simulink model "Simulacion_stepper"  (R2025b)
settings: Solver=ode4  StartTime=0.0  StopTime=Time_simulation  FixedStep=1/frecuency_simulation  RelTol=1e-3
InitFcn:
  | %%InitFcn();
StopFcn:
  | %%FinishFcn
model workspace (MAT data in the model file):
  Ts_stepper = 0.001
values from neighbouring files (symbols this model uses):
  B = motor_params.B_internal    [bode.m]    (also in current_observer.m = 0.0005; discretizacion.m = [ 1/L, 0; ekf_4_estados.m = params.B; obs_ctrl_back_emf_ext.m = [1/L 0)
  frecuency_simulation = 10e3    (= 10000)    [InitFcn.m]
  J = motor_params.J_internal    [bode.m]    (also in current_observer.m = 0.008; ekf_4_estados.m = params.J; obs_ctrl_back_emf_ext.m = 0.008; obs_y_contrl_back_emd.m = 0.008)
  Ke = 0.0055    [current_observer.m]    (also in ekf_4_estados.m = params.Ke; observer.m = Pvec(3); salient_motor.m = 0.0066)
  Ki_d = PI_dq_params.Ki_d_salient    [bode.m]
  Ki_q = PI_dq_params.Ki_q_salient    [bode.m]
  Ki_w = (wn_w^2)*J_var/Kt    [Barrido_B.m]    (also in Barrido_J.m; bode.m = PI_MTPA_params.Ki_w)
  Kp_d = PI_dq_params.Kp_d_salient    [bode.m]
  Kp_q = PI_dq_params.Kp_q_salient    [bode.m]
  Kp_w = (2*shi_w*wn_w*J_var)/Kt    [Barrido_B.m]    (also in Barrido_J.m; bode.m = PI_MTPA_params.Kp_w)
  Kt = Nr*Ke    (= 0.275)    [current_observer.m]    (also in ekf_4_estados.m = params.Kt; frecuencia_max.m = 0.33; observer.m = Pvec(4); salient_motor.m = 0.33)
  L = place(A', C', 10*eig(A)).'    [current_observer.m]    (also in desfase.m = lags(k); discretizacion.m = 0.01; frecuencia_max.m = 0.006; obs_ctrl_back_emf_ext.m = 0.006)
  P = motor_params.P    [bode.m]    (also in ekf_4_estados.m = P_pred; frecuencia_max.m = 50; salient_motor.m = 50)
  R = motor_params.R    [bode.m]    (also in current_observer.m = 3.4; discretizacion.m = 3.4; ekf_4_estados.m = params.R; frecuencia_max.m = 3.4)
  sample_time = 1/frecuency_simulation    (= 0.0001)    [InitFcn.m]
  Ts_current = 1/f_current    (= 0.0001)    [InitFcn.m]
  Ts_Wm = Ts_current*10    (= 0.001)    [InitFcn.m]
  Vdc = 24    [InitFcn.m]    (also in frecuencia_max.m = 12)
undefined symbols (not defined in the file or in its folder): DiscIntNeverNeededParam, EKF_params, motor_params, RI_base
libraries: simulink x8, mcbeeMathTransformLib x3, spspowerguiLib x1
(part 2 of 5)

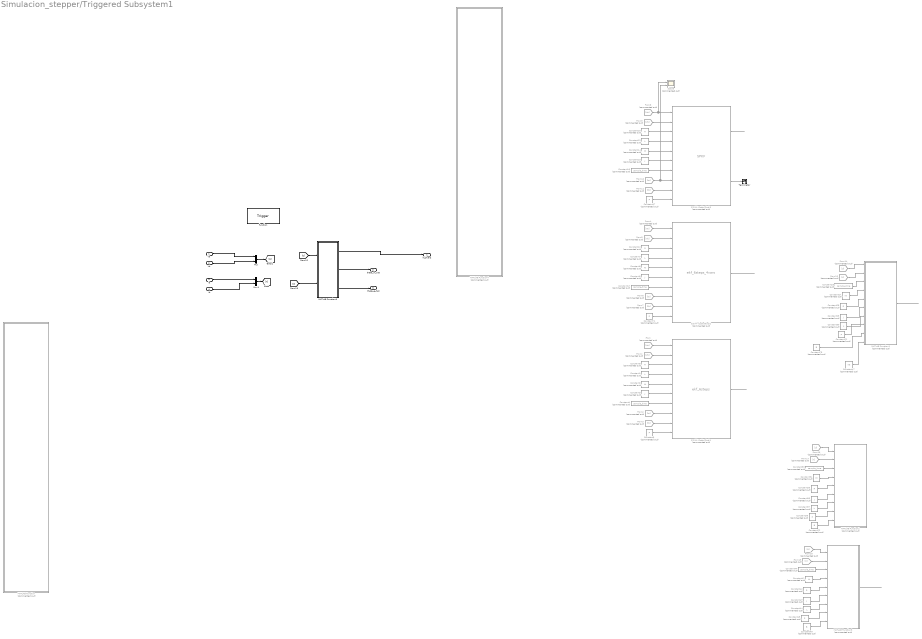
== system Simulacion_stepper/Triggered Subsystem1 ==
  Va : Inport
  Vb : Inport  Port=2
  Ia : Inport  Port=3
  Ib : Inport  Port=4
  function : TriggerPort  TriggerType=function-call  VariantControl=(inherit)  SampleTime=1/100
  C/C++ Code Block1 : S-Function  Commented=on  FunctionName=ekf_6steps  SFunctionModules=ekf_6steps_wrapper.c  SFunctionDeploymentMode=off  EnableBusSupport=off  mask(S-Function Builder){}
      mask help: Simulink:masks:SFunctionBuilder_MD
      mask init: same as Simulacion_stepper/Motor 1  Speed PR/C/C++ Code Block
      settings: CopyFcn=set_param(gcbh,'LinkStatus','none')  OpenFcn=sfunctionwizard(gcbh)
      mask Display:
      | plot(val(:,1),val(:,2))
      | disp(sys)
      | port_label('input',1,sprintf('%s', 'Va'),'interpreter','tex')
      | port_label('input',2,sprintf('%s', 'Vb'),'interpreter','tex')
      | port_label('input',3,sprintf('%s', 'R'),'interpreter','tex')
      | port_label('input',4,sprintf('%s', 'L'),'interpreter','tex')
      | port_label('input',5,sprintf('%s', 'Kt'),'interpreter','tex')
      | port_label('input',6,sprintf('%s', 'J'),'interpreter','tex')
      | port_label('input',7,sprintf('%s', 'Ts'),'interpreter','tex')
      | port_label('input',8,sprintf('%s', 'Ia\_medido'),'interpreter','tex')
      | port_label('input',9,sprintf('%s', 'Ib\_medido'),'interpreter','tex')
      | port_label('input',10,sprintf('%s', 'Nr'),'interpreter','tex')
      | port_label('output',1,sprintf('%s', 'x\_corr\_out'),'interpreter','tex')
  C/C++ Code Block2 : S-Function  Commented=on  FunctionName=ekf_6steps_4vars  SFunctionModules=ekf_6steps_4vars_wrapper.c  SFunctionDeploymentMode=off  EnableBusSupport=off  mask(S-Function Builder){}
      mask help: Simulink:masks:SFunctionBuilder_MD
      mask init: same as Simulacion_stepper/Motor 1  Speed PR/C/C++ Code Block
      settings: CopyFcn=set_param(gcbh,'LinkStatus','none')  OpenFcn=sfunctionwizard(gcbh)
      mask Display:
      | plot(val(:,1),val(:,2))
      | disp(sys)
      | port_label('input',1,sprintf('%s', 'Va'),'interpreter','tex')
      | port_label('input',2,sprintf('%s', 'Vb'),'interpreter','tex')
      | port_label('input',3,sprintf('%s', 'R'),'interpreter','tex')
      | port_label('input',4,sprintf('%s', 'L'),'interpreter','tex')
      | port_label('input',5,sprintf('%s', 'Kt'),'interpreter','tex')
      | port_label('input',6,sprintf('%s', 'J'),'interpreter','tex')
      | port_label('input',7,sprintf('%s', 'Ts'),'interpreter','tex')
      | port_label('input',8,sprintf('%s', 'Ia\_medido'),'interpreter','tex')
      | port_label('input',9,sprintf('%s', 'Ib\_medido'),'interpreter','tex')
      | port_label('input',10,sprintf('%s', 'Nr'),'interpreter','tex')
      | port_label('output',1,sprintf('%s', 'x\_corr\_out'),'interpreter','tex')
  C/C++ Code Block3 : S-Function  Commented=on  FunctionName=SPKF  SFunctionModules=SPKF_wrapper.c  SFunctionDeploymentMode=off  EnableBusSupport=off  mask(S-Function Builder){}
      mask help: Simulink:masks:SFunctionBuilder_MD
      mask init: same as Simulacion_stepper/Motor 1  Speed PR/C/C++ Code Block
      settings: CopyFcn=set_param(gcbh,'LinkStatus','none')  OpenFcn=sfunctionwizard(gcbh)
      mask Display:
      | plot(val(:,1),val(:,2))
      | disp(sys)
      | port_label('input',1,sprintf('%s', 'Va'),'interpreter','tex')
      | port_label('input',2,sprintf('%s', 'Vb'),'interpreter','tex')
      | port_label('input',3,sprintf('%s', 'R'),'interpreter','tex')
      | port_label('input',4,sprintf('%s', 'L'),'interpreter','tex')
      | port_label('input',5,sprintf('%s', 'Kt'),'interpreter','tex')
      | port_label('input',6,sprintf('%s', 'J'),'interpreter','tex')
      | port_label('input',7,sprintf('%s', 'Ts'),'interpreter','tex')
      | port_label('input',8,sprintf('%s', 'Ia\_medido'),'interpreter','tex')
      | port_label('input',9,sprintf('%s', 'Ib\_medido'),'interpreter','tex')
      | port_label('input',10,sprintf('%s', 'Nr'),'interpreter','tex')
      | port_label('output',1,sprintf('%s', 'x'),'interpreter','tex')
      | port_label('output',2,sprintf('%s', 'x\_aux'),'interpreter','tex')
  Constant{1,7,13,30,37,44} (6 alike) : Constant  Commented=on  Value=L  OutDataTypeStr=double
  Constant{4,10,16,26,33,40} (6 alike) : Constant  Commented=on  Value=sample_time  OutDataTypeStr=double
  Constant{5,11,17,31,38,45} (6 alike) : Constant  Commented=on  Value=P  OutDataTypeStr=double
  Constant{6,12,18,28,35,42} (6 alike) : Constant  Commented=on  Value=R  OutDataTypeStr=double
  Constant{2,8,14,27,34,41} (6 alike) : Constant  Commented=on  Value=Kt  OutDataTypeStr=double
  Constant{3,9,15,29,36,43} (6 alike) : Constant  Commented=on  Value=J  OutDataTypeStr=double
  Constant25 : Constant  Commented=on  Value=B
  Constant32 : Constant  Commented=on  Value=B
  Constant39 : Constant  Commented=on  Value=B
  Constant47 : Constant  Commented=on  Value=Ke  OutDataTypeStr=double
  From : From  Commented=on  GotoTag=Va
  From1 : From  Commented=on  GotoTag=Vb
  From10 : From  Commented=on  GotoTag=Ia
  From11 : From  Commented=on  GotoTag=Ib
  From14 : From  Commented=on  GotoTag=U
  From15 : From  Commented=on  GotoTag=X
  From16 : From  Commented=on  GotoTag=U
  From17 : From  Commented=on  GotoTag=X
  From18 : From  Commented=on  GotoTag=U
  From19 : From  Commented=on  GotoTag=X
  From2 : From  Commented=on  GotoTag=Ia
  From3 : From  Commented=on  GotoTag=Ib
  From4 : From  Commented=on  GotoTag=Va
  From5 : From  Commented=on  GotoTag=Vb
  From6 : From  Commented=on  GotoTag=Ia
  From7 : From  Commented=on  GotoTag=Ib
  From8 : From  Commented=on  GotoTag=Va
  From9 : From  Commented=on  GotoTag=Vb
  MATLAB Function : MATLAB Function  Commented=on  TreatAsAtomicUnit=on
  MATLAB Function1 : MATLAB Function  Commented=on  TreatAsAtomicUnit=on
  MATLAB Function2 : MATLAB Function  Commented=on  TreatAsAtomicUnit=on
  MATLAB Function3 : MATLAB Function  Commented=on  TreatAsAtomicUnit=on
  MATLAB Function4 : MATLAB Function  Commented=on  TreatAsAtomicUnit=on
  MATLAB Function5 : MATLAB Function  TreatAsAtomicUnit=on
  Mux : Mux  Inputs=2
  Mux1 : Mux  Inputs=2
  Scope : Scope  Commented=on  NumInputPorts=2
      settings: ActiveDisplayYMinimum=-25.65057  ActiveDisplayYMaximum=25.22013
  Terminator : Terminator
  kf_5var2 : Outport  PortDimensions=[5 1]
  theta_m_hat : Outport  Port=2
  theta_e_hat : Outport  Port=3
  wires:
  Constant4/1 -> C/C++ Code Block1/7
  Constant5/1 -> C/C++ Code Block1/10
  C/C++ Code Block1/1 -> ?
  Constant6/1 -> C/C++ Code Block1/3
  Constant1/1 -> C/C++ Code Block1/4
  Constant2/1 -> C/C++ Code Block1/5
  Constant3/1 -> C/C++ Code Block1/6
  C/C++ Code Block2/1 -> ?
  C/C++ Code Block3/1 -> ?
  Vb/1 -> Mux/2
  Va/1 -> Mux/1
  Ib/1 -> Mux1/2
  Ia/1 -> Mux1/1
  From/1 -> C/C++ Code Block1/1
  From1/1 -> C/C++ Code Block1/2
  From2/1 -> C/C++ Code Block1/8
  From3/1 -> C/C++ Code Block1/9
  From4/1 -> C/C++ Code Block2/1
  From7/1 -> C/C++ Code Block2/9
  Constant8/1 -> C/C++ Code Block2/5
  Constant12/1 -> C/C++ Code Block2/3
  From5/1 -> C/C++ Code Block2/2
  Constant11/1 -> C/C++ Code Block2/10
  From6/1 -> C/C++ Code Block2/8
  Constant9/1 -> C/C++ Code Block2/6
  Constant7/1 -> C/C++ Code Block2/4
  Constant10/1 -> C/C++ Code Block2/7
  From8/1 -> Scope/1, C/C++ Code Block3/1
  From11/1 -> C/C++ Code Block3/9
  Constant14/1 -> C/C++ Code Block3/5
  Constant18/1 -> C/C++ Code Block3/3
  From9/1 -> C/C++ Code Block3/2
  Constant17/1 -> C/C++ Code Block3/10
  From10/1 -> Scope/2, C/C++ Code Block3/8
  Constant15/1 -> C/C++ Code Block3/6
  Constant13/1 -> C/C++ Code Block3/4
  Constant16/1 -> C/C++ Code Block3/7
  C/C++ Code Block3/2 -> Terminator/1
  Mux1/1 -> [X]
  Mux/1 -> [U]
  From16/1 -> MATLAB Function2/1(U)
  From17/1 -> MATLAB Function2/2(Y)
  Constant33/1 -> MATLAB Function2/3(Ts)
  Constant32/1 -> MATLAB Function2/9(B)
  Constant37/1 -> MATLAB Function2/7(L)
  Constant35/1 -> MATLAB Function2/5(R)
  Constant36/1 -> MATLAB Function2/6(J)
  Constant34/1 -> MATLAB Function2/4(Kt)
  Constant38/1 -> MATLAB Function2/8(Nr)
  MATLAB Function3/1(x_corr) -> ?
  Constant45/1 -> MATLAB Function3/8(Nr)
  Constant41/1 -> MATLAB Function3/4(Kt)
  From19/1 -> MATLAB Function3/2(Y)
  Constant43/1 -> MATLAB Function3/6(J)
  Constant40/1 -> MATLAB Function3/3(Ts)
  Constant39/1 -> MATLAB Function3/9(B)
  Constant42/1 -> MATLAB Function3/5(R)
  From18/1 -> MATLAB Function3/1(U)
  Constant44/1 -> MATLAB Function3/7(L)
  From15/1 -> MATLAB Function1/2(X)
  Constant27/1 -> MATLAB Function1/4(Kt)
  Constant31/1 -> MATLAB Function1/8(Nr)
  Constant29/1 -> MATLAB Function1/6(J)
  Constant25/1 -> MATLAB Function1/9(B)
  Constant26/1 -> MATLAB Function1/3(Ts)
  Constant30/1 -> MATLAB Function1/7(L)
  Constant28/1 -> MATLAB Function1/5(R)
  From14/1 -> MATLAB Function1/1(U)
  Constant47/1 -> MATLAB Function1/10(Ke)
  MATLAB Function1/1(x_corr) -> ?
  [X] -> MATLAB Function5/2(X)
  [U] -> MATLAB Function5/1(U)
  MATLAB Function5/1(x_out) -> kf_5var2/1
  MATLAB Function5/2(theta_m_hat) -> theta_m_hat/1
  MATLAB Function5/3(theta_e_out) -> theta_e_hat/1

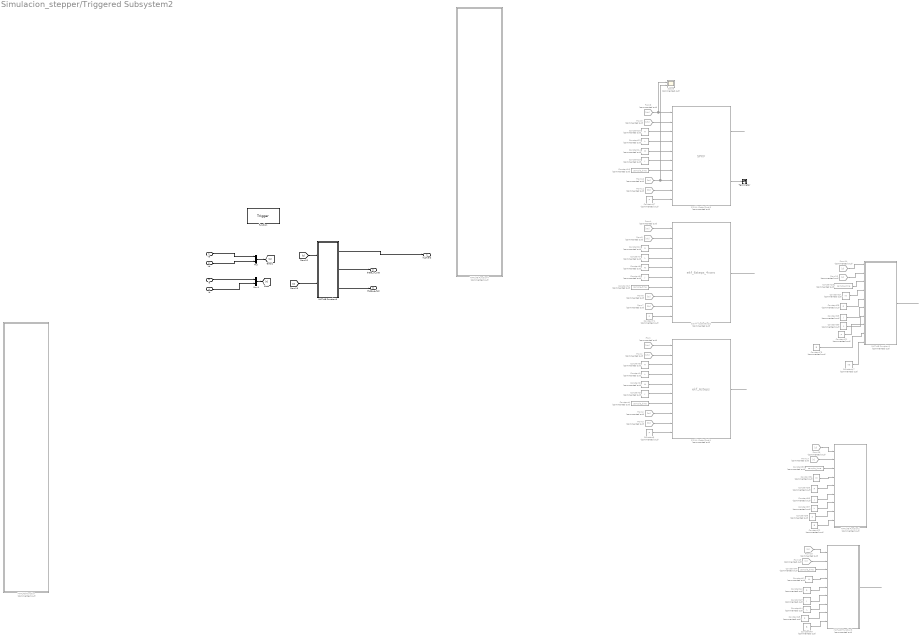
== system Simulacion_stepper/Triggered Subsystem2 ==
  Va : Inport
  Vb : Inport  Port=2
  Ia : Inport  Port=3
  Ib : Inport  Port=4
  function : TriggerPort  TriggerType=function-call  VariantControl=(inherit)  SampleTime=1/100
  C/C++ Code Block1 : S-Function  Commented=on  FunctionName=ekf_6steps  SFunctionModules=ekf_6steps_wrapper.c  SFunctionDeploymentMode=off  EnableBusSupport=off  mask(S-Function Builder){}
      mask help: Simulink:masks:SFunctionBuilder_MD
      mask init: same as Simulacion_stepper/Motor 1  Speed PR/C/C++ Code Block
      settings: CopyFcn=set_param(gcbh,'LinkStatus','none')  OpenFcn=sfunctionwizard(gcbh)
      mask Display:
      | plot(val(:,1),val(:,2))
      | disp(sys)
      | port_label('input',1,sprintf('%s', 'Va'),'interpreter','tex')
      | port_label('input',2,sprintf('%s', 'Vb'),'interpreter','tex')
      | port_label('input',3,sprintf('%s', 'R'),'interpreter','tex')
      | port_label('input',4,sprintf('%s', 'L'),'interpreter','tex')
      | port_label('input',5,sprintf('%s', 'Kt'),'interpreter','tex')
      | port_label('input',6,sprintf('%s', 'J'),'interpreter','tex')
      | port_label('input',7,sprintf('%s', 'Ts'),'interpreter','tex')
      | port_label('input',8,sprintf('%s', 'Ia\_medido'),'interpreter','tex')
      | port_label('input',9,sprintf('%s', 'Ib\_medido'),'interpreter','tex')
      | port_label('input',10,sprintf('%s', 'Nr'),'interpreter','tex')
      | port_label('output',1,sprintf('%s', 'x\_corr\_out'),'interpreter','tex')
  C/C++ Code Block2 : S-Function  Commented=on  FunctionName=ekf_6steps_4vars  SFunctionModules=ekf_6steps_4vars_wrapper.c  SFunctionDeploymentMode=off  EnableBusSupport=off  mask(S-Function Builder){}
      mask help: Simulink:masks:SFunctionBuilder_MD
      mask init: same as Simulacion_stepper/Motor 1  Speed PR/C/C++ Code Block
      settings: CopyFcn=set_param(gcbh,'LinkStatus','none')  OpenFcn=sfunctionwizard(gcbh)
      mask Display:
      | plot(val(:,1),val(:,2))
      | disp(sys)
      | port_label('input',1,sprintf('%s', 'Va'),'interpreter','tex')
      | port_label('input',2,sprintf('%s', 'Vb'),'interpreter','tex')
      | port_label('input',3,sprintf('%s', 'R'),'interpreter','tex')
      | port_label('input',4,sprintf('%s', 'L'),'interpreter','tex')
      | port_label('input',5,sprintf('%s', 'Kt'),'interpreter','tex')
      | port_label('input',6,sprintf('%s', 'J'),'interpreter','tex')
      | port_label('input',7,sprintf('%s', 'Ts'),'interpreter','tex')
      | port_label('input',8,sprintf('%s', 'Ia\_medido'),'interpreter','tex')
      | port_label('input',9,sprintf('%s', 'Ib\_medido'),'interpreter','tex')
      | port_label('input',10,sprintf('%s', 'Nr'),'interpreter','tex')
      | port_label('output',1,sprintf('%s', 'x\_corr\_out'),'interpreter','tex')
  C/C++ Code Block3 : S-Function  Commented=on  FunctionName=SPKF  SFunctionModules=SPKF_wrapper.c  SFunctionDeploymentMode=off  EnableBusSupport=off  mask(S-Function Builder){}
      mask help: Simulink:masks:SFunctionBuilder_MD
      mask init: same as Simulacion_stepper/Motor 1  Speed PR/C/C++ Code Block
      settings: CopyFcn=set_param(gcbh,'LinkStatus','none')  OpenFcn=sfunctionwizard(gcbh)
      mask Display:
      | plot(val(:,1),val(:,2))
      | disp(sys)
      | port_label('input',1,sprintf('%s', 'Va'),'interpreter','tex')
      | port_label('input',2,sprintf('%s', 'Vb'),'interpreter','tex')
      | port_label('input',3,sprintf('%s', 'R'),'interpreter','tex')
      | port_label('input',4,sprintf('%s', 'L'),'interpreter','tex')
      | port_label('input',5,sprintf('%s', 'Kt'),'interpreter','tex')
      | port_label('input',6,sprintf('%s', 'J'),'interpreter','tex')
      | port_label('input',7,sprintf('%s', 'Ts'),'interpreter','tex')
      | port_label('input',8,sprintf('%s', 'Ia\_medido'),'interpreter','tex')
      | port_label('input',9,sprintf('%s', 'Ib\_medido'),'interpreter','tex')
      | port_label('input',10,sprintf('%s', 'Nr'),'interpreter','tex')
      | port_label('output',1,sprintf('%s', 'x'),'interpreter','tex')
      | port_label('output',2,sprintf('%s', 'x\_aux'),'interpreter','tex')
  Constant{1,7,13,30,37,44} (6 alike) : Constant  Commented=on  Value=L  OutDataTypeStr=double
  Constant{4,10,16,26,33,40} (6 alike) : Constant  Commented=on  Value=sample_time  OutDataTypeStr=double
  Constant{5,11,17,31,38,45} (6 alike) : Constant  Commented=on  Value=P  OutDataTypeStr=double
  Constant{6,12,18,28,35,42} (6 alike) : Constant  Commented=on  Value=R  OutDataTypeStr=double
  Constant{2,8,14,27,34,41} (6 alike) : Constant  Commented=on  Value=Kt  OutDataTypeStr=double
  Constant{3,9,15,29,36,43} (6 alike) : Constant  Commented=on  Value=J  OutDataTypeStr=double
  Constant25 : Constant  Commented=on  Value=B
  Constant32 : Constant  Commented=on  Value=B
  Constant39 : Constant  Commented=on  Value=B
  Constant47 : Constant  Commented=on  Value=Ke  OutDataTypeStr=double
  From : From  Commented=on  GotoTag=Va
  From1 : From  Commented=on  GotoTag=Vb
  From10 : From  Commented=on  GotoTag=Ia
  From11 : From  Commented=on  GotoTag=Ib
  From14 : From  Commented=on  GotoTag=U
  From15 : From  Commented=on  GotoTag=X
  From16 : From  Commented=on  GotoTag=U
  From17 : From  Commented=on  GotoTag=X
  From18 : From  Commented=on  GotoTag=U
  From19 : From  Commented=on  GotoTag=X
  From2 : From  Commented=on  GotoTag=Ia
  From3 : From  Commented=on  GotoTag=Ib
  From4 : From  Commented=on  GotoTag=Va
  From5 : From  Commented=on  GotoTag=Vb
  From6 : From  Commented=on  GotoTag=Ia
  From7 : From  Commented=on  GotoTag=Ib
  From8 : From  Commented=on  GotoTag=Va
  From9 : From  Commented=on  GotoTag=Vb
  MATLAB Function : MATLAB Function  Commented=on  TreatAsAtomicUnit=on
  MATLAB Function1 : MATLAB Function  Commented=on  TreatAsAtomicUnit=on
  MATLAB Function2 : MATLAB Function  Commented=on  TreatAsAtomicUnit=on
  MATLAB Function3 : MATLAB Function  Commented=on  TreatAsAtomicUnit=on
  MATLAB Function4 : MATLAB Function  Commented=on  TreatAsAtomicUnit=on
  MATLAB Function5 : MATLAB Function  TreatAsAtomicUnit=on
  Mux : Mux  Inputs=2
  Mux1 : Mux  Inputs=2
  Scope : Scope  Commented=on  NumInputPorts=2
      settings: ActiveDisplayYMinimum=-25.65057  ActiveDisplayYMaximum=25.22013
  Terminator : Terminator
  kf_5var2 : Outport  PortDimensions=[5 1]
  theta_m_hat : Outport  Port=2
  theta_e_hat : Outport  Port=3
  wires:
  Constant4/1 -> C/C++ Code Block1/7
  Constant5/1 -> C/C++ Code Block1/10
  C/C++ Code Block1/1 -> ?
  Constant6/1 -> C/C++ Code Block1/3
  Constant1/1 -> C/C++ Code Block1/4
  Constant2/1 -> C/C++ Code Block1/5
  Constant3/1 -> C/C++ Code Block1/6
  C/C++ Code Block2/1 -> ?
  C/C++ Code Block3/1 -> ?
  Vb/1 -> Mux/2
  Va/1 -> Mux/1
  Ib/1 -> Mux1/2
  Ia/1 -> Mux1/1
  From/1 -> C/C++ Code Block1/1
  From1/1 -> C/C++ Code Block1/2
  From2/1 -> C/C++ Code Block1/8
  From3/1 -> C/C++ Code Block1/9
  From4/1 -> C/C++ Code Block2/1
  From7/1 -> C/C++ Code Block2/9
  Constant8/1 -> C/C++ Code Block2/5
  Constant12/1 -> C/C++ Code Block2/3
  From5/1 -> C/C++ Code Block2/2
  Constant11/1 -> C/C++ Code Block2/10
  From6/1 -> C/C++ Code Block2/8
  Constant9/1 -> C/C++ Code Block2/6
  Constant7/1 -> C/C++ Code Block2/4
  Constant10/1 -> C/C++ Code Block2/7
  From8/1 -> Scope/1, C/C++ Code Block3/1
  From11/1 -> C/C++ Code Block3/9
  Constant14/1 -> C/C++ Code Block3/5
  Constant18/1 -> C/C++ Code Block3/3
  From9/1 -> C/C++ Code Block3/2
  Constant17/1 -> C/C++ Code Block3/10
  From10/1 -> Scope/2, C/C++ Code Block3/8
  Constant15/1 -> C/C++ Code Block3/6
  Constant13/1 -> C/C++ Code Block3/4
  Constant16/1 -> C/C++ Code Block3/7
  C/C++ Code Block3/2 -> Terminator/1
  Mux1/1 -> [X]
  Mux/1 -> [U]
  From16/1 -> MATLAB Function2/1(U)
  From17/1 -> MATLAB Function2/2(Y)
  Constant33/1 -> MATLAB Function2/3(Ts)
  Constant32/1 -> MATLAB Function2/9(B)
  Constant37/1 -> MATLAB Function2/7(L)
  Constant35/1 -> MATLAB Function2/5(R)
  Constant36/1 -> MATLAB Function2/6(J)
  Constant34/1 -> MATLAB Function2/4(Kt)
  Constant38/1 -> MATLAB Function2/8(Nr)
  MATLAB Function3/1(x_corr) -> ?
  Constant45/1 -> MATLAB Function3/8(Nr)
  Constant41/1 -> MATLAB Function3/4(Kt)
  From19/1 -> MATLAB Function3/2(Y)
  Constant43/1 -> MATLAB Function3/6(J)
  Constant40/1 -> MATLAB Function3/3(Ts)
  Constant39/1 -> MATLAB Function3/9(B)
  Constant42/1 -> MATLAB Function3/5(R)
  From18/1 -> MATLAB Function3/1(U)
  Constant44/1 -> MATLAB Function3/7(L)
  From15/1 -> MATLAB Function1/2(X)
  Constant27/1 -> MATLAB Function1/4(Kt)
  Constant31/1 -> MATLAB Function1/8(Nr)
  Constant29/1 -> MATLAB Function1/6(J)
  Constant25/1 -> MATLAB Function1/9(B)
  Constant26/1 -> MATLAB Function1/3(Ts)
  Constant30/1 -> MATLAB Function1/7(L)
  Constant28/1 -> MATLAB Function1/5(R)
  From14/1 -> MATLAB Function1/1(U)
  Constant47/1 -> MATLAB Function1/10(Ke)
  MATLAB Function1/1(x_corr) -> ?
  [X] -> MATLAB Function5/2(X)
  [U] -> MATLAB Function5/1(U)
  MATLAB Function5/1(x_out) -> kf_5var2/1
  MATLAB Function5/2(theta_m_hat) -> theta_m_hat/1
  MATLAB Function5/3(theta_e_out) -> theta_e_hat/1

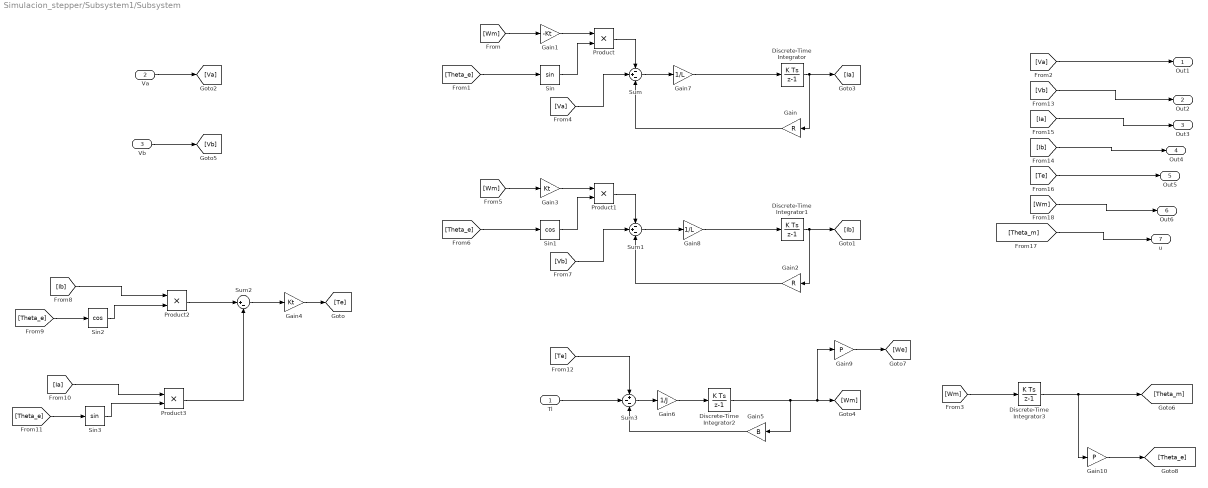
== system Simulacion_stepper/Subsystem1/Subsystem ==
  Tl : Inport
  Va : Inport  Port=2
  Vb : Inport  Port=3
  Discrete-Time Integrator{,1..3} (4 alike) : DiscreteIntegrator  SampleTime=sample_time  ICPrevOutput=DiscIntNeverNeededParam  ICPrevScaledInput=DiscIntNeverNeededParam
  Gain : Gain  Gain=R
  Gain1 : Gain  Gain=-Kt
  Gain10 : Gain  Gain=P
  Gain2 : Gain  Gain=R
  Gain3 : Gain  Gain=Kt
  Gain4 : Gain  Gain=Kt
  Gain5 : Gain  Gain=B
  Gain6 : Gain  Gain=1/J
  Gain7 : Gain  Gain=1/L
  Gain8 : Gain  Gain=1/L
  Gain9 : Gain  Gain=P
  Product{,1..3} (4 alike) : Product
  Sin : Trigonometry
  Sin1 : Trigonometry  Operator=cos
  Sin2 : Trigonometry  Operator=cos
  Sin3 : Trigonometry
  Sum : Sum  Inputs=-+-
  Sum1 : Sum  Inputs=-+-
  Sum2 : Sum  Inputs=|+-
  Sum3 : Sum  Inputs=+--
  Out1 : Outport
  Out2 : Outport  Port=2
  Out3 : Outport  Port=3
  Out4 : Outport  Port=4
  Out5 : Outport  Port=5
  Out6 : Outport  Port=6
  u : Outport  Port=7
  wires:
  Discrete-Time Integrator/1 -> [Ia], Gain/1
  Discrete-Time Integrator2/1 -> Gain5/1, Gain9/1, [Wm]
  [Wm] -> Discrete-Time Integrator3/1
  [Vb] -> Out2/1
  [Ia] -> Out3/1
  [Ib] -> Out4/1
  [Te] -> Out5/1
  [Wm] -> Out6/1
  [Theta_m] -> u/1
  [Va] -> Out1/1
  Discrete-Time Integrator3/1 -> Gain10/1, [Theta_m]
  Vb/1 -> [Vb]
  Va/1 -> [Va]
  [Wm] -> Gain1/1
  Gain1/1 -> Product/1
  Sin/1 -> Product/2
  [Theta_e] -> Sin/1
  Product/1 -> Sum/1
  [Va] -> Sum/2
  Gain/1 -> Sum/3
  Gain2/1 -> Sum1/3
  [Wm] -> Gain3/1
  [Vb] -> Sum1/2
  [Theta_e] -> Sin1/1
  Gain3/1 -> Product1/1
  Sin1/1 -> Product1/2
  Discrete-Time Integrator1/1 -> [Ib], Gain2/1
  Product1/1 -> Sum1/1
  [Ib] -> Product2/1
  Sin2/1 -> Product2/2
  [Theta_e] -> Sin2/1
  [Ia] -> Product3/1
  [Theta_e] -> Sin3/1
  Sin3/1 -> Product3/2
  Product2/1 -> Sum2/1
  Product3/1 -> Sum2/2
  Sum2/1 -> Gain4/1
  Gain4/1 -> [Te]
  [Te] -> Sum3/1
  Tl/1 -> Sum3/2
  Gain5/1 -> Sum3/3
  Sum3/1 -> Gain6/1
  Sum/1 -> Gain7/1
  Gain7/1 -> Discrete-Time Integrator/1
  Sum1/1 -> Gain8/1
  Gain8/1 -> Discrete-Time Integrator1/1
  Gain6/1 -> Discrete-Time Integrator2/1
  Gain9/1 -> [We]
  Gain10/1 -> [Theta_e]

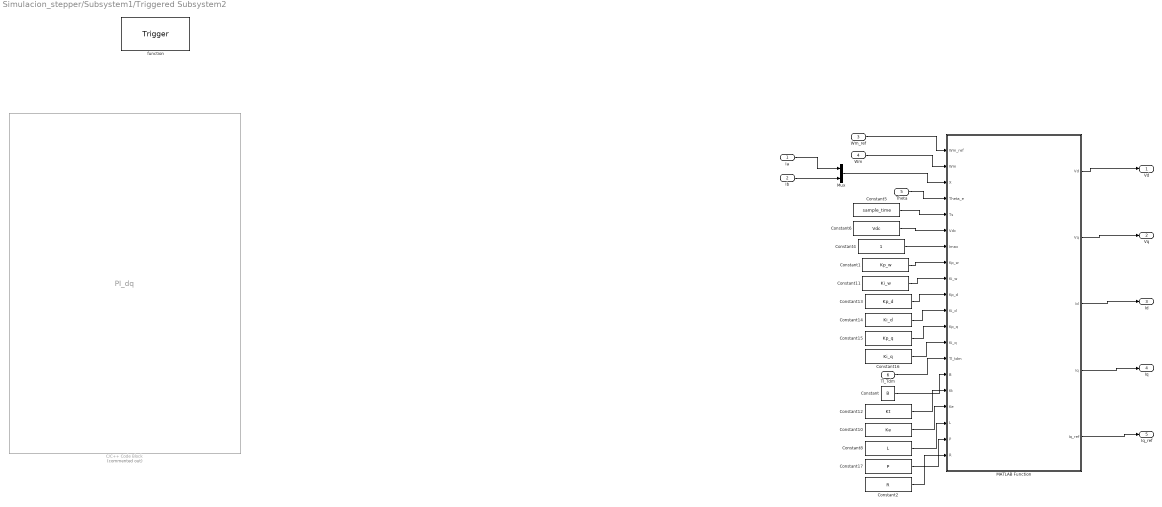
== system Simulacion_stepper/Subsystem1/Triggered Subsystem2 ==
  Ia : Inport
  Ib : Inport  Port=2
  Wm_ref : Inport  Port=3
  Wm : Inport  Port=4
  Theta : Inport  Port=5
  Tl_Tdm : Inport  Port=6
  function : TriggerPort  TriggerType=function-call  VariantControl=(inherit)  SampleTime=1/100
  C/C++ Code Block : S-Function  Commented=on  FunctionName=PI_dq  SFunctionModules=PI_dq_wrapper.c  SFunctionDeploymentMode=off  EnableBusSupport=off  mask(S-Function Builder){}
      mask help: Simulink:masks:SFunctionBuilder_MD
      mask init: same as Simulacion_stepper/Motor 1  Speed PR/C/C++ Code Block
      settings: CopyFcn=set_param(gcbh,'LinkStatus','none')  OpenFcn=sfunctionwizard(gcbh)
      mask Display:
      | plot(val(:,1),val(:,2))
      | disp(sys)
      | port_label('input',1,sprintf('%s', 'Ia'),'interpreter','tex')
      | port_label('input',2,sprintf('%s', 'Ib'),'interpreter','tex')
      | port_label('input',3,sprintf('%s', 'Wm\_ref'),'interpreter','tex')
      | port_label('input',4,sprintf('%s', 'Wm\_ext'),'interpreter','tex')
      | port_label('input',5,sprintf('%s', 'Kp\_current'),'interpreter','tex')
      | port_label('input',6,sprintf('%s', 'Ki\_current'),'interpreter','tex')
      | port_label('input',7,sprintf('%s', 'Kd\_current'),'interpreter','tex')
      | port_label('input',8,sprintf('%s', 'sample\_time\_ext'),'interpreter','tex')
      | port_label('input',9,sprintf('%s', 'Vdc\_ext'),'interpreter','tex')
      | port_label('input',10,sprintf('%s', 'R\_ext'),'interpreter','tex')
      | port_label('input',11,sprintf('%s', 'Ld\_ext'),'interpreter','tex')
      | port_label('input',12,sprintf('%s', 'Lq\_ext'),'interpreter','tex')
      | port_label('input',13,sprintf('%s', 'Ke\_ext'),'interpreter','tex')
      | port_label('input',14,sprintf('%s', 'Theta\_ext'),'interpreter','tex')
      | port_label('input',15,sprintf('%s', 'Kp\_wm'),'interpreter','tex')
      | port_label('input',16,sprintf('%s', 'Ki\_wm'),'interpreter','tex')
      | port_label('input',17,sprintf('%s', 'Tl\_Tdm'),'interpreter','tex')
      | port_label('input',18,sprintf('%s', 'B'),'interpreter','tex')
      | port_label('input',19,sprintf('%s', 'Kt\_ext'),'interpreter','tex')
      | port_label('output',1,sprintf('%s', 'Ud'),'interpreter','tex')
      | port_label('output',2,sprintf('%s', 'Uq'),'interpreter','tex')
      | port_label('output',3,sprintf('%s', 'Id'),'interpreter','tex')
      | port_label('output',4,sprintf('%s', 'Iq'),'interpreter','tex')
      | port_label('output',5,sprintf('%s', 'Iq\_ref\_aux'),'interpreter','tex')
  Constant : Constant  Value=B  OutDataTypeStr=double
  Constant1 : Constant  Value=Kp_w  OutDataTypeStr=double
  Constant10 : Constant  Value=Ke  OutDataTypeStr=double
  Constant11 : Constant  Value=Ki_w  OutDataTypeStr=double
  Constant12 : Constant  Value=Kt  OutDataTypeStr=double
  Constant13 : Constant  Value=Kp_d  OutDataTypeStr=double
  Constant14 : Constant  Value=Ki_d  OutDataTypeStr=double
  Constant15 : Constant  Value=Kp_q  OutDataTypeStr=double
  Constant16 : Constant  Value=Ki_q  OutDataTypeStr=double
  Constant17 : Constant  Value=P  OutDataTypeStr=double
  Constant2 : Constant  Value=R  OutDataTypeStr=double
  Constant4 : Constant  OutDataTypeStr=double
  Constant5 : Constant  Value=sample_time  OutDataTypeStr=double
  Constant6 : Constant  Value=Vdc  OutDataTypeStr=double
  Constant8 : Constant  Value=L  OutDataTypeStr=double
  MATLAB Function : MATLAB Function  TreatAsAtomicUnit=on
  Mux : Mux  Inputs=2
  Vd : Outport
  Vq : Outport  Port=2
  Id : Outport  Port=3
  Iq : Outport  Port=4
  Iq_ref : Outport  Port=5
  wires:
  MATLAB Function/1(Vd) -> Vd/1
  MATLAB Function/2(Vq) -> Vq/1
  MATLAB Function/3(Id) -> Id/1
  MATLAB Function/4(Iq) -> Iq/1
  MATLAB Function/5(Iq_ref) -> Iq_ref/1
  Wm_ref/1 -> MATLAB Function/1(Wm_ref)
  Wm/1 -> MATLAB Function/2(Wm)
  Ia/1 -> Mux/1
  Ib/1 -> Mux/2
  Mux/1 -> MATLAB Function/3(X)
  Theta/1 -> MATLAB Function/4(Theta_e)
  Constant5/1 -> MATLAB Function/5(Ts)
  Constant6/1 -> MATLAB Function/6(Vdc)
  Constant12/1 -> MATLAB Function/16(Kt)
  Constant/1 -> MATLAB Function/15(B)
  Tl_Tdm/1 -> MATLAB Function/14(Tl_tdm)
  Constant1/1 -> MATLAB Function/8(Kp_w)
  Constant11/1 -> MATLAB Function/9(Ki_w)
  Constant13/1 -> MATLAB Function/10(Kp_d)
  Constant14/1 -> MATLAB Function/11(Ki_d)
  Constant15/1 -> MATLAB Function/12(Kp_q)
  Constant16/1 -> MATLAB Function/13(Ki_q)
  Constant10/1 -> MATLAB Function/17(Ke)
  Constant8/1 -> MATLAB Function/18(L)
  Constant17/1 -> MATLAB Function/19(P)
  Constant4/1 -> MATLAB Function/7(Imax)
  Constant2/1 -> MATLAB Function/20(R)

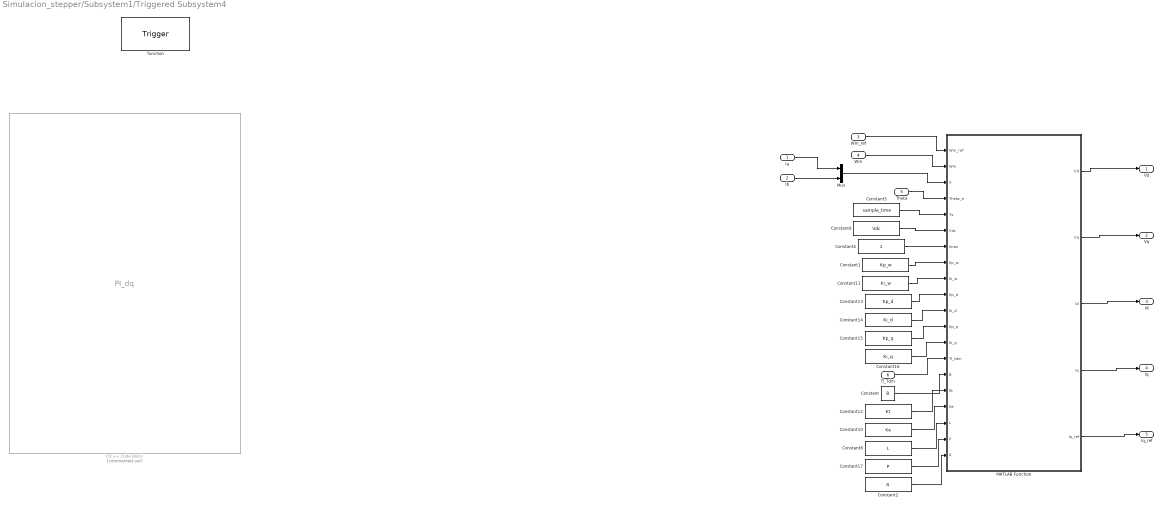
== system Simulacion_stepper/Subsystem1/Triggered Subsystem4 ==
  Ia : Inport
  Ib : Inport  Port=2
  Wm_ref : Inport  Port=3
  Wm : Inport  Port=4
  Theta : Inport  Port=5
  Tl_Tdm : Inport  Port=6
  function : TriggerPort  TriggerType=function-call  VariantControl=(inherit)  SampleTime=1/100
  C/C++ Code Block : S-Function  Commented=on  FunctionName=PI_dq  SFunctionModules=PI_dq_wrapper.c  SFunctionDeploymentMode=off  EnableBusSupport=off  mask(S-Function Builder){}
      mask help: Simulink:masks:SFunctionBuilder_MD
      mask init: same as Simulacion_stepper/Motor 1  Speed PR/C/C++ Code Block
      settings: CopyFcn=set_param(gcbh,'LinkStatus','none')  OpenFcn=sfunctionwizard(gcbh)
      mask Display:
      | plot(val(:,1),val(:,2))
      | disp(sys)
      | port_label('input',1,sprintf('%s', 'Ia'),'interpreter','tex')
      | port_label('input',2,sprintf('%s', 'Ib'),'interpreter','tex')
      | port_label('input',3,sprintf('%s', 'Wm\_ref'),'interpreter','tex')
      | port_label('input',4,sprintf('%s', 'Wm\_ext'),'interpreter','tex')
      | port_label('input',5,sprintf('%s', 'Kp\_current'),'interpreter','tex')
      | port_label('input',6,sprintf('%s', 'Ki\_current'),'interpreter','tex')
      | port_label('input',7,sprintf('%s', 'Kd\_current'),'interpreter','tex')
      | port_label('input',8,sprintf('%s', 'sample\_time\_ext'),'interpreter','tex')
      | port_label('input',9,sprintf('%s', 'Vdc\_ext'),'interpreter','tex')
      | port_label('input',10,sprintf('%s', 'R\_ext'),'interpreter','tex')
      | port_label('input',11,sprintf('%s', 'Ld\_ext'),'interpreter','tex')
      | port_label('input',12,sprintf('%s', 'Lq\_ext'),'interpreter','tex')
      | port_label('input',13,sprintf('%s', 'Ke\_ext'),'interpreter','tex')
      | port_label('input',14,sprintf('%s', 'Theta\_ext'),'interpreter','tex')
      | port_label('input',15,sprintf('%s', 'Kp\_wm'),'interpreter','tex')
      | port_label('input',16,sprintf('%s', 'Ki\_wm'),'interpreter','tex')
      | port_label('input',17,sprintf('%s', 'Tl\_Tdm'),'interpreter','tex')
      | port_label('input',18,sprintf('%s', 'B'),'interpreter','tex')
      | port_label('input',19,sprintf('%s', 'Kt\_ext'),'interpreter','tex')
      | port_label('output',1,sprintf('%s', 'Ud'),'interpreter','tex')
      | port_label('output',2,sprintf('%s', 'Uq'),'interpreter','tex')
      | port_label('output',3,sprintf('%s', 'Id'),'interpreter','tex')
      | port_label('output',4,sprintf('%s', 'Iq'),'interpreter','tex')
      | port_label('output',5,sprintf('%s', 'Iq\_ref\_aux'),'interpreter','tex')
  Constant : Constant  Value=B  OutDataTypeStr=double
  Constant1 : Constant  Value=Kp_w  OutDataTypeStr=double
  Constant10 : Constant  Value=Ke  OutDataTypeStr=double
  Constant11 : Constant  Value=Ki_w  OutDataTypeStr=double
  Constant12 : Constant  Value=Kt  OutDataTypeStr=double
  Constant13 : Constant  Value=Kp_d  OutDataTypeStr=double
  Constant14 : Constant  Value=Ki_d  OutDataTypeStr=double
  Constant15 : Constant  Value=Kp_q  OutDataTypeStr=double
  Constant16 : Constant  Value=Ki_q  OutDataTypeStr=double
  Constant17 : Constant  Value=P  OutDataTypeStr=double
  Constant2 : Constant  Value=R  OutDataTypeStr=double
  Constant4 : Constant  OutDataTypeStr=double
  Constant5 : Constant  Value=sample_time  OutDataTypeStr=double
  Constant6 : Constant  Value=Vdc  OutDataTypeStr=double
  Constant8 : Constant  Value=L  OutDataTypeStr=double
  MATLAB Function : MATLAB Function  TreatAsAtomicUnit=on
  Mux : Mux  Inputs=2
  Vd : Outport
  Vq : Outport  Port=2
  Id : Outport  Port=3
  Iq : Outport  Port=4
  Iq_ref : Outport  Port=5
  wires:
  MATLAB Function/1(Vd) -> Vd/1
  MATLAB Function/2(Vq) -> Vq/1
  MATLAB Function/3(Id) -> Id/1
  MATLAB Function/4(Iq) -> Iq/1
  MATLAB Function/5(Iq_ref) -> Iq_ref/1
  Wm_ref/1 -> MATLAB Function/1(Wm_ref)
  Wm/1 -> MATLAB Function/2(Wm)
  Ia/1 -> Mux/1
  Ib/1 -> Mux/2
  Mux/1 -> MATLAB Function/3(X)
  Theta/1 -> MATLAB Function/4(Theta_e)
  Constant5/1 -> MATLAB Function/5(Ts)
  Constant6/1 -> MATLAB Function/6(Vdc)
  Constant12/1 -> MATLAB Function/16(Kt)
  Constant/1 -> MATLAB Function/15(B)
  Tl_Tdm/1 -> MATLAB Function/14(Tl_tdm)
  Constant1/1 -> MATLAB Function/8(Kp_w)
  Constant11/1 -> MATLAB Function/9(Ki_w)
  Constant13/1 -> MATLAB Function/10(Kp_d)
  Constant14/1 -> MATLAB Function/11(Ki_d)
  Constant15/1 -> MATLAB Function/12(Kp_q)
  Constant16/1 -> MATLAB Function/13(Ki_q)
  Constant10/1 -> MATLAB Function/17(Ke)
  Constant8/1 -> MATLAB Function/18(L)
  Constant17/1 -> MATLAB Function/19(P)
  Constant4/1 -> MATLAB Function/7(Imax)
  Constant2/1 -> MATLAB Function/20(R)

== matlab function Simulacion_stepper/Triggered Subsystem1/MATLAB Function1 ==
  data: U input; x_corr output; X input; Ts input; Kt input; R input; J input; L input; Nr input; B input; Ke input
function x_corr = ekf_5var(U,X,Ts,Kt,R,J,L,Nr,B,Ke)
persistent x_hat P x_pred
%%  x_hat son los estados predichos
%%  x_corr es la salida corregida
%%  P_pre ó Sum_less es la covarianza predicha
%%  P ó sum_more es la covarianza
%%  Rk ó sum_v es la covarianza de incertidumbre del sensor




 %%Iniciamos calculando X_hat[k-1]
 if isempty(x_hat)
     x_hat = zeros(5,1);
     P = diag([1e-4 1e-4 1e-6 1e-10 1e-4]);
     x_corr = zeros(5,1);
     x_pred = zeros(5,1);


 end

Qk = diag([1e-4 1e-4 1e-4 1e-10 1e-6]);
Rk = diag([5e-4 5e-4]);   % ruido de medición

%%1A
%%Predicción
Ia = x_hat(1);
Ib = x_hat(2);
Wm = x_hat(3);
Th_m = x_hat(4);
Tx = x_hat(5);

Th_e = Nr*Th_m;
S = sin(Th_e);
C = cos(Th_e);

Va = U(1);
Vb = U(2);

dx = zeros(5,1);
dx(1) = (Va - R*Ia + Ke*Wm*S)/L;
dx(2) = (Vb - R*Ib - Ke*Wm*C)/L;
dx(3) = (Kt*(Ib*C-Ia*S) -Tx)/J;
dx(4) = Wm;
dx(5) = 0;
x_pred = x_hat + Ts*dx;
x_pred(4) = wrap_2pi(x_pred(4));

%%Calculamos el jacobiano
RL = R/L;
uno = Ke*S;
dos = Ke*C;

A = [-RL 0   (uno/L) (dos*Nr*Wm/L) 0;
 0  -RL   -dos/L    uno*Nr*Wm/L  0;
 -uno/J dos/J -1/J -Kt*Nr*(Ia*C+Ib*S)/J -1/J;
 0 0 1 0 0;
 0 0 0 0 0];

A_hat = eye(5) + Ts*A;
A_hat_T = transpose(A_hat);

%%1B COVARIANZA PREDICHA
P_pred = A_hat * P * A_hat_T + Qk; 


%%1C PREDECIMOS LA SALIDA DEL SISTEMA
Ck = [1 0 0 0 0;
      0 1 0 0 0];
Ck_T = transpose(Ck);
y_pred = Ck*x_pred;

%%2A calculamos la matriz Lk
%%Lk = P_pred *Ck_T * inv(Ck*P_pred*Ck_T + sum_v)
Sk = Ck*P_pred*Ck_T + Rk;
Lk = P_pred * Ck_T /Sk;

%%2B Actualizamos los estados estados corregidos en función de L


y_meas = [X(1);X(2)];

innov = y_meas - y_pred;
x_corr = x_pred + Lk*(innov);
x_corr(4) = wrap_2pi(x_corr(4));
%%actualizamos la covarianza y guardamos el estado
x_hat = x_corr;
Lk_T = transpose(Lk);
P = P_pred - Lk*Sk*Lk_T;
P_T = transpose(P);
P = 0.5 * (P + P_T);

== matlab function Simulacion_stepper/MATLAB Function4 ==
  data: u input; y output
function y = fcn(u)

y = wrap_2pi(u);

== matlab function Simulacion_stepper/Triggered Subsystem1/MATLAB Function2 ==
  data: U input size=2; x_corr output; Y input size=2; Ts input; Kt input; R input; J input; L input; Nr input; B input
function x_corr = SPKF_4var(U,Y,Ts,Kt,R,J,L,Nr,B)
persistent x_hat P  alpham alphac Qk Rk h
%%  x_hat son los estados predichos
%%  x_corr es la salida corregida
%%  P_pre ó Sum_less es la covarianza predicha
%%  P ó sum_more es la covarianza
%%  Rk ó sum_v es la covarianza de incertidumbre del sensor


Nx = 4; %%Números de estados
Nw = 4; %% Incertidumbres de estado
Ny = 2; %% Incertidumbre de mediciones
Na = Nx+Nw+Ny;


%%Los métodos de sigma-point pueden diferir al utilizar las variables
%%alpha. Existen 2 métodos:

%% Método |    Sigma       |     alpha_m_0      | alpha_m_k         |           alpha_c_0               | alpha_c_k |
%% UKF    | sqrt(L+lambda) |  lambda/(L+Lambda) | 1/(2*(L+Lambda))  | alpha_m_0 + (1-alpha^2 + betha)   | alpha_m_k |
%% CDKF   |    h           |   (h^2 - L)/h^2    |  1/(2*h^2)        | alpha_m_0                         | alpha_m_k |
 %%Iniciamos calculando X_hat[k-1]
 if isempty(x_hat)
    
     %%Utilizamos el CDKF, con h = sqrt(Nxa); 
        x_hat = zeros(Nx,1);
        h =sqrt(Na);
        alpham = ones(2*Na+1,1) * (1/(2*h^2));
        alpham(1) = (h^2 - Na)/(h^2);   % peso del sigma central
        alphac = alpham;             
     %%Valores de covarianza
     P = diag([1e-2 1e-2 1e-6 1e-12 ]);
     Qk = diag([1e-2 1e-2 1e-8 1e-12 ]);
     Rk = [1e-4 0; 0 1e-4];
 end
    
     x_corr = zeros(Nx,1);
     x_pred = zeros(Nx,1);
     x_hat_a = zeros(Na,1);
     X_minus = zeros(Nx,2*Na+1);
     Y_minus = zeros(Ny,2*Na+1);
%%Ciclo de 2*Na+1
%%Aun que deberiamos hacer un ciclo for, en matlab se hace solo asi que no
%%es necesario

%% 1A-I Creamos el vector de estados extendidos
x_hat_a = [x_hat;zeros(Nw,1);zeros(Ny,1)]; 


%% 1A-II Conseguimos el factor de cholesky


%%Creamos la matriz de covarianza extendidas, el cual es de la forma
%%             [P   0    0]
%%     P_a =   [0   Qk   0]
%%             [0   0   Rk]

P_a = blkdiag(P,Qk,Rk);
Sa = chol(P_a,"lower");

%% 1A-III generamos los sigma points
%% Queda de la forma [x_hat_a, x_hat_a + h*S,x_hat_a - h*S] (Por eso es 2*Nxa+1 = N)
%% Al usar x_a x_a(:,ones(1,Na)) creamos una matriz de la forma [x_a,x_a...x_a], que es de tamaño (Na)x(2*Na+1)
%% Posteriormente, se le suma un vector de [0,+h*S,-h*S]
%% Cómo S es del tamaño (Nxa)x(Nxa), el total es de (2*Na+1 = N)
X =  x_hat_a(:,ones(1,2*Na+1)) + h*[zeros(Na,1), Sa, -Sa];

%% 1A-IV Calculamos las ecuaciones de estado
Va = U(1);
Vb = U(2);


for k=1:2*Na+1

  % --- separar estado, ruido de proceso y ruido de medición ---


xk = X(1:Nx,k);                     % [Ia; Ib; Wm; Th_m]
wk = X(Nx+1 : Nx+Nw,k);             % ruido de proceso (4x1)
vk = X(Nx+Nw+1 : end,k);            % ruido de medición (2x1)    

Ia = xk(1);
Ib = xk(2);
Wm = xk(3);
Th_m = xk(4);

Th_e = Nr*Th_m;
S = sin(Th_e);
C = cos(Th_e);


dx1 = (Va - R*Ia + Kt*Wm*S)/L;
dx2 = (Vb - R*Ib - Kt*Wm*C)/L;
dx3 = (Kt*(Ib*C-Ia*S)-B*Wm)/J;
dx4 = Wm;

%Calculamos el paso siguiente mediante euler
%% X_minus corresponde a la matriz que contiene todos los sigma-points distribuidos en los estados del sistema no-extendido (Nx)x(Na)
X_minus(1,k) = Ia + Ts*dx1+ wk(1);
X_minus(2,k) = Ib + Ts*dx2 + wk(2);
X_minus(3,k) = Wm + Ts*dx3 + wk(3);
X_minus(4,k) = Th_m + Ts*dx4 + wk(4);
%%X_minus(4,k) = wrap_2pi(X_minus(4,k));

Y_minus(1,k) = X_minus(1,k) + vk(1);
Y_minus(2,k) = X_minus(2,k) + vk(2);

end
%% 1B Reconstrucción de la media
%% Esta matriz contiene la media de todos los estados. (Nx)x(1)
x_pred = X_minus*alpham;
y_pred = Y_minus*alpham;
%%  Reconstrucción de la covarianza

%% Acá lo que hacemos es copiar la media N veces, para poder realizar la resta.
%%Pero realmente debería ser un for de [Xs(i,k)= X_minus(i,k) - x_pred(i)],
%%dónde K es cada variable de estado (Nx)
%% Xs es una matriz de desviación respecto a la media. Es necesario para construir la covarianza P
Xs = X_minus - x_pred(:,ones([1 2*Na+1])); 
Ys = Y_minus - y_pred(:,ones([1 2*Na+1]));

Xs_T = transpose(Xs);
Ys_T = transpose(Ys);
%%Calculamos la matriz de covarianza, pero hay que considerar que como
%%diag(alphac) es una matriz llena de diagonales, uno puede reducir la
%%cantidad de cómputo.
P_pred = Xs*diag(alphac)*Xs_T;
Pyy = Ys* diag(alphac)* Ys_T;
Pxy = Xs*diag(alphac)*Ys_T;
Lk = Pxy/Pyy;
Lk_T = transpose(Lk);
%% 2B Leemos la medición y actualizamos
x_corr = x_pred + Lk*(Y - y_pred);
x_corr(4) = wrap_2pi(x_corr(4));
%%Guardamos los valores de x_hat para mantenerlos
x_hat = x_corr; 
%% 2C Actualizamos la covarianza
P = P_pred - Lk*Pyy*Lk_T;
P_T = transpose(P);
P = 0.5 * (P + P_T);

== matlab function Simulacion_stepper/Triggered Subsystem1/MATLAB Function3 ==
  data: U input size=2; x_corr output; Y input size=2; Ts input; Kt input; R input; J input; L input; Nr input; B input
function x_corr = SPKF_5var(U,Y,Ts,Kt,R,J,L,Nr,B)
persistent x_hat P x_pred alpham alphac Qk Rk h
%%  x_hat son los estados predichos
%%  x_corr es la salida corregida
%%  P_pre ó Sum_less es la covarianza predicha
%%  P ó sum_more es la covarianza
%%  Rk ó sum_v es la covarianza de incertidumbre del sensor


Nx = 5; %%Números de estados
Nw = 5; %% Incertidumbres de estado
Ny = 2; %% Incertidumbre de mediciones
Na = Nx+Nw+Ny;


%%Los métodos de sigma-point pueden diferir al utilizar las variables
%%alpha. Existen 2 métodos:

%% Método |    Sigma       |     alpha_m_0      | alpha_m_k         |           alpha_c_0               | alpha_c_k |
%% UKF    | sqrt(L+lambda) |  lambda/(L+Lambda) | 1/(2*(L+Lambda))  | alpha_m_0 + (1-alpha^2 + betha)   | alpha_m_k |
%% CDKF   |    h           |   (h^2 - L)/h^2    |  1/(2*h^2)        | alpha_m_0                         | alpha_m_k |
 %%Iniciamos calculando X_hat[k-1]
 if isempty(x_hat)
    
     %%Utilizamos el CDKF, con h = sqrt(Nxa); 
        x_hat = zeros(Nx,1);
        h =sqrt(Na);
        alpham = ones(2*Na+1,1) * (1/(2*h^2));
        alpham(1) = (h^2 - Na)/(h^2);   % peso del sigma central
        alphac = alpham;             
     %%Valores de covarianza
     P = diag([1e-2 1e-2 1e-4 1e-8 1e-12]);
     Qk = diag([1e-2 1e-2 1e-6 1e-8 1e-12]);
     Rk = [1e-4 0; 0 1e-4];
 end
    
     x_corr = zeros(Nx,1);
     x_pred = zeros(Nx,1);
     x_hat_a = zeros(Na,1);
     X_minus = zeros(Nx,2*Na+1);
     Y_minus = zeros(Ny,2*Na+1);
%%Ciclo de 2*Na+1
%%Aun que deberiamos hacer un ciclo for, en matlab se hace solo asi que no
%%es necesario

%% 1A-I Creamos el vector de estados extendidos
x_hat_a = [x_hat;zeros(Nw,1);zeros(Ny,1)]; 


%% 1A-II Conseguimos el factor de cholesky


%%Creamos la matriz de covarianza extendidas, el cual es de la forma
%%             [P   0    0]
%%     P_a =   [0   Qk   0]
%%             [0   0   Rk]

P_a = blkdiag(P,Qk,Rk);
Sa = chol(P_a,"lower");

%% 1A-III generamos los sigma points
%% Queda de la forma [x_hat_a, x_hat_a + h*S,x_hat_a - h*S] (Por eso es 2*Nxa+1 = N)
%% Al usar x_a x_a(:,ones(1,Na)) creamos una matriz de la forma [x_a,x_a...x_a], que es de tamaño (Na)x(2*Na+1)
%% Posteriormente, se le suma un vector de [0,+h*S,-h*S]
%% Cómo S es del tamaño (Nxa)x(Nxa), el total es de (2*Na+1 = N)
X =  x_hat_a(:,ones(1,2*Na+1)) + h*[zeros(Na,1), Sa, -Sa];

%% 1A-IV Calculamos las ecuaciones de estado
Va = U(1);
Vb = U(2);


for k=1:2*Na+1

  % --- separar estado, ruido de proceso y ruido de medición ---


xk = X(1:Nx,k);                     % [Ia; Ib; Wm; Th_m]
wk = X(Nx+1 : Nx+Nw,k);             % ruido de proceso (4x1)
vk = X(Nx+Nw+1 : end,k);            % ruido de medición (2x1)    

Ia = xk(1);
Ib = xk(2);
Wm = xk(3);
Th_m = xk(4);
Tx = xk(5);

Th_e = Nr*Th_m;
S = sin(Th_e);
C = cos(Th_e);


dx1 = (Va - R*Ia + Kt*Wm*S)/L;
dx2 = (Vb - R*Ib - Kt*Wm*C)/L;
dx3 = (Kt*(Ib*C-Ia*S)-B*Wm - Tx)/J;
dx4 = Wm;
dTx = 0;

%Calculamos el paso siguiente mediante euler
%% X_minus corresponde a la matriz que contiene todos los sigma-points distribuidos en los estados del sistema no-extendido (Nx)x(Na)
X_minus(1,k) = Ia + Ts*dx1+ wk(1);
X_minus(2,k) = Ib + Ts*dx2 + wk(2);
X_minus(3,k) = Wm + Ts*dx3 + wk(3);
X_minus(4,k) = Th_m + Ts*dx4 + wk(4);
X_minus(4,k) = wrap_2pi(X_minus(4,k));
X_minus(5,k) = Tx + Ts*dTx + wk(5);

Y_minus(1,k) = X_minus(1,k) + vk(1);
Y_minus(2,k) = X_minus(2,k) + vk(2);

end
%% 1B Reconstrucción de la media
%% Esta matriz contiene la media de todos los estados. (Nx)x(1)
x_pred = X_minus*alpham;
y_pred = Y_minus*alpham;
%%  Reconstrucción de la covarianza

%% Acá lo que hacemos es copiar la media N veces, para poder realizar la resta.
%%Pero realmente debería ser un for de [Xs(i,k)= X_minus(i,k) - x_pred(i)],
%%dónde K es cada variable de estado (Nx)
%% Xs es una matriz de desviación respecto a la media. Es necesario para construir la covarianza P
Xs = X_minus - x_pred(:,ones([1 2*Na+1])); 
Ys = Y_minus - y_pred(:,ones([1 2*Na+1]));

Xs_T = transpose(Xs);
Ys_T = transpose(Ys);
%%Calculamos la matriz de covarianza, pero hay que considerar que como
%%diag(alphac) es una matriz llena de diagonales, uno puede reducir la
%%cantidad de cómputo.
P_pred = Xs*diag(alphac)*Xs_T;
Pyy = Ys* diag(alphac)* Ys_T;
Pxy = Xs*diag(alphac)*Ys_T;
Lk = Pxy/Pyy;
Lk_T = transpose(Lk);
%% 2B Leemos la medición y actualizamos
x_corr = x_pred + Lk*(Y - y_pred);
x_corr(4) = wrap_2pi(x_corr(4));
%%Guardamos los valores de x_hat para mantenerlos
x_hat = x_corr; 
%% 2C Actualizamos la covarianza
P = P_pred - Lk*Pyy*Lk_T;
P_T = transpose(P);
P = 0.5 * (P + P_T);
